simulink model "Q1"  (R2018b)
settings: Solver=VariableStepAuto  StartTime=0.0  StopTime=10.0  RelTol=1e-3
settings Model: Creator=N.GH  LastModifiedBy=N.GH

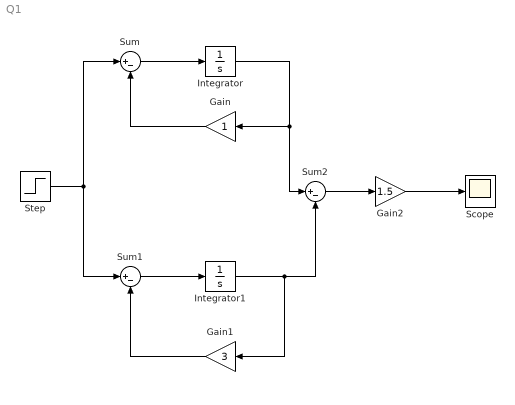
== system Q1 ==
  Gain : Gain
  Gain1 : Gain  Gain=3
  Gain2 : Gain  Gain=1.5
  Integrator : Integrator
  Integrator1 : Integrator
  Scope : Scope
  Step : Step  SampleTime=0
  Sum : Sum  Inputs=|+-
  Sum1 : Sum  Inputs=|+-
  Sum2 : Sum  Inputs=|+-
  wires:
  Step/1 -> Sum/1, Sum1/1
  Gain/1 -> Sum/2
  Sum/1 -> Integrator/1
  Integrator/1 -> Sum2/1, Gain/1
  Integrator1/1 -> Sum2/2, Gain1/1
  Sum1/1 -> Integrator1/1
  Gain1/1 -> Sum1/2
  Sum2/1 -> Gain2/1
  Gain2/1 -> Scope/1
